simulink model "filter_realize"  (R2020a)
settings: Solver=VariableStepAuto  StartTime=0.0  StopTime=10.0  RelTol=1e-3
model workspace (MAT data in the model file):
  A = 0.4
  B = 0.5
  C = -0.25
settings Model: Creator=007  LastModifiedBy=007

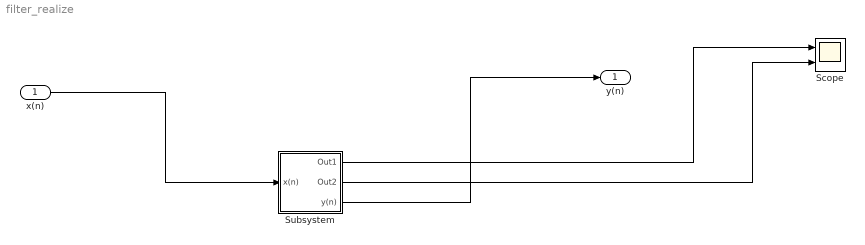
== system filter_realize ==
  x(n) : Inport
  Scope : Scope  NumInputPorts=2
  Subsystem : Subsystem
  y(n) : Outport
  wires:
  x(n)/1 -> Subsystem/1(x(n))
  Subsystem/1(Out1) -> Scope/1
  Subsystem/2(Out2) -> Scope/2
  Subsystem/3(y(n)) -> y(n)/1

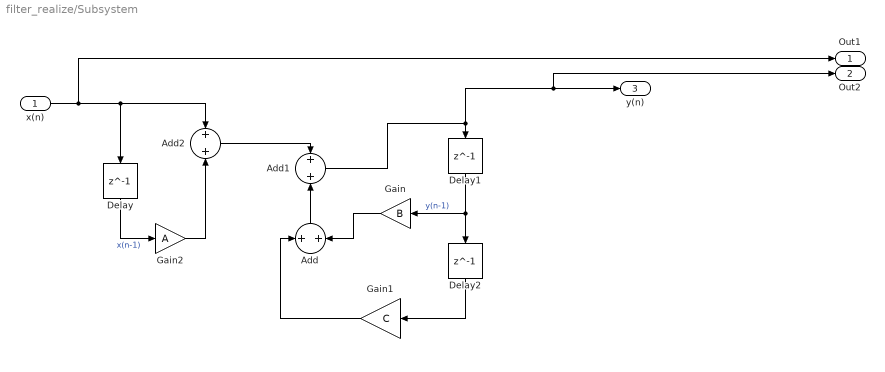
== system filter_realize/Subsystem ==
  x(n) : Inport
  Add : Sum
  Add1 : Sum
  Add2 : Sum
  Delay : Delay  DelayLength=1
  Delay1 : Delay  DelayLength=1
  Delay2 : Delay  DelayLength=1
  Gain : Gain  Gain=B
  Gain1 : Gain  Gain=C
  Gain2 : Gain  Gain=A
  Out1 : Outport
  Out2 : Outport  Port=2
  y(n) : Outport  Port=3
  wires:
  Add1/1 -> y(n)/1, Out2/1, Delay1/1
  Gain/1 -> Add/2
  Add/1 -> Add1/2
  Delay/1 -> Gain2/1  "x(n-1)"
  Gain1/1 -> Add/1
  Add2/1 -> Add1/1
  x(n)/1 -> Out1/1, Add2/1, Delay/1
  Delay1/1 -> Delay2/1, Gain/1  "y(n-1)"
  Delay2/1 -> Gain1/1
  Gain2/1 -> Add2/2
